simulink model "problem3"  (R2020b)
settings: Solver=VariableStepAuto  StartTime=0.0  StopTime=120  RelTol=1e-3
model workspace (MAT data in the model file):
  b = Simulink.Parameter
  b.Value = 50
  b.DataType = 'auto'
  b.Dimensions = [1 1]
  m = Simulink.Parameter
  m.Value = 1000
  m.DataType = 'auto'
  m.Dimensions = [1 1]
  u = Simulink.Parameter
  u.Value = 500
  u.DataType = 'auto'
  u.Dimensions = [1 1]
values from neighbouring files (symbols this model uses):
  b = 50.0    [CC_data.sldd]
  m = 1000.0    [CC_data.sldd]
settings Model: Creator=Varun  LastModifiedBy=Varun

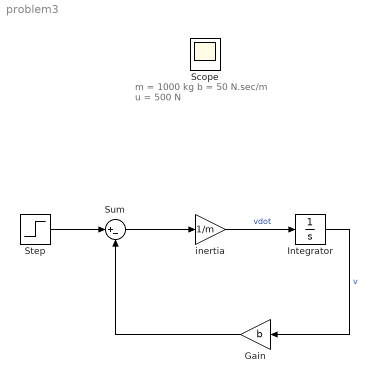
== system problem3 ==
  note: m = 1000 kg
      | b = 50 N.sec/m
      | u = 500 N
  Gain : Gain  Gain=b
  Integrator : Integrator
  Step : Step  Time=0  After=u  SampleTime=0
  Sum : Sum  Inputs=|+-
  inertia : Gain  Gain=1/m
  Scope : Scope
  wires:
  Gain/1 -> Sum/2
  Sum/1 -> inertia/1
  inertia/1 -> Integrator/1  "vdot"
  Integrator/1 -> Gain/1  "v"
  Step/1 -> Sum/1
